simulink model "ACC_Main"  (R2025a)
settings: Solver=VariableStepAuto  StopTime=30
PostLoadFcn:
  | accRoot = fileparts(get_param('ACC_Main','FileName'));
  | addpath(accRoot, fullfile(accRoot,'models'), fullfile(accRoot,'scripts'));
  | run(fullfile(accRoot,'scripts','acc_init_setup.m'));
  | clear accRoot
undefined symbols (not defined in the file): D_followBlend_m, D_safe, k_closing
settings Model: Creator=Quang Huy  LastModifiedBy=ASUS
settings DebuggingCC: UnconnectedInputMsg=warning  UnconnectedOutputMsg=warning  UnconnectedLineMsg=warning

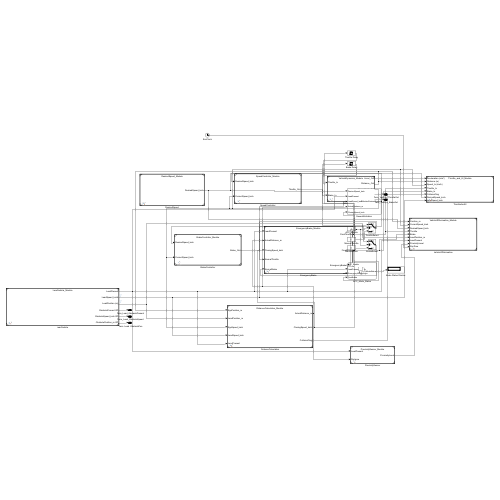
[thumbnail: Simulink's stored preview of the top-level diagram]
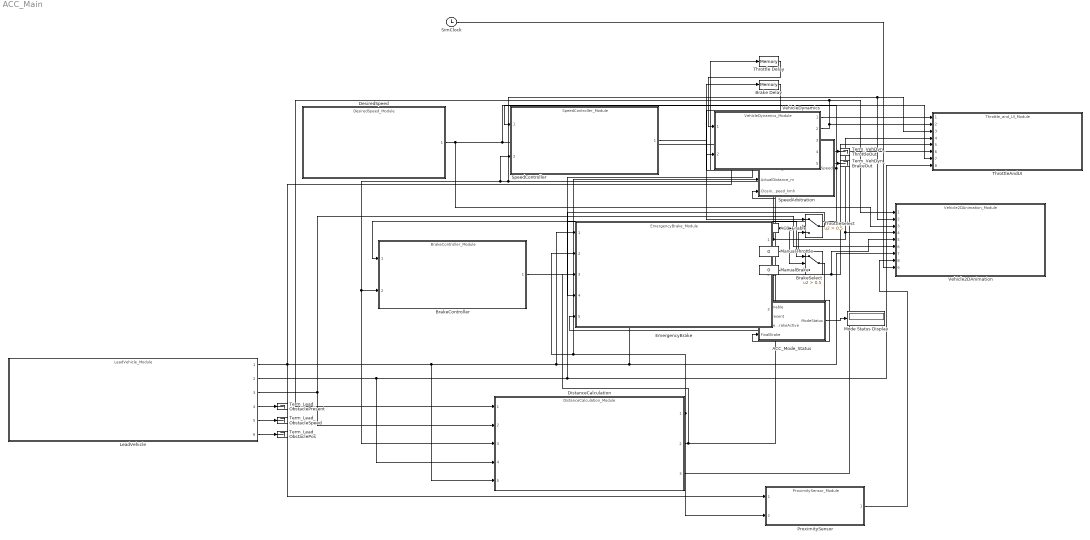
== system ACC_Main ==
  ACC_Enable : Constant  OutDataTypeStr=boolean
  ACC_Mode_Status : Stateflow chart  TreatAsAtomicUnit=on
  Brake Delay : Memory
  BrakeController : ModelReference  ModelNameDialog=BrakeController_Module.slx  SimulationMode=Normal  ModelReferenceVersion=3.0
  BrakeSelect : Switch  Criteria=u2 > Threshold  Threshold=0.5  SaturateOnIntegerOverflow=off  InputSameDT=off
  DesiredSpeed : ModelReference  ModelNameDialog=DesiredSpeed_Module.slx  SimulationMode=Normal  ModelReferenceVersion=3.0
  DistanceCalculation : ModelReference  ModelNameDialog=DistanceCalculation_Module.slx  SimulationMode=Normal  ModelReferenceVersion=3.0
  EmergencyBrake : ModelReference  ModelNameDialog=EmergencyBrake_Module.slx  SimulationMode=Normal  ModelReferenceVersion=3.0
  LeadVehicle : ModelReference  ModelNameDialog=LeadVehicle_Module.slx  SimulationMode=Normal  ModelReferenceVersion=3.2
  ManualBrake : Constant  Value=0
  ManualThrottle : Constant  Value=0  OutDataTypeStr=double
  Mode Status Display : Display
  ProximitySensor : ModelReference  ModelNameDialog=ProximitySensor_Module.slx  SimulationMode=Normal  ModelReferenceVersion=1.2
  SimClock : Clock
  SpeedArbitration : Subsystem
  SpeedController : ModelReference  ModelNameDialog=SpeedController_Module.slx  SimulationMode=Normal  ModelReferenceVersion=3.0
  Term_Lead_ObstaclePos : Terminator
  Term_Lead_ObstaclePresent : Terminator
  Term_Lead_ObstacleSpeed : Terminator
  Term_VehDyn_BrakeOut : Terminator
  Term_VehDyn_ThrottleOut : Terminator
  Throttle Delay : Memory
  ThrottleAndUI : ModelReference  ModelNameDialog=Throttle_and_UI_Module.slx  SimulationMode=Normal  ModelReferenceVersion=3.2
  ThrottleSelect : Switch  Criteria=u2 > Threshold  Threshold=0.5  SaturateOnIntegerOverflow=off  InputSameDT=off
  Vehicle2DAnimation : ModelReference  ModelNameDialog=Vehicle2DAnimation_Module.slx  SimulationMode=Normal  ModelReferenceVersion=3.1
  VehicleDynamics : ModelReference  ModelNameDialog=VehicleDynamics_Module.slx  SimulationMode=Normal  ModelReferenceVersion=3.0
  wires:
  DesiredSpeed/1 -> SpeedArbitration/1(DesiredSpeed_kmh), ThrottleAndUI/7, Vehicle2DAnimation/3
  LeadVehicle/3 -> DistanceCalculation/2, Vehicle2DAnimation/6
  LeadVehicle/2 -> SpeedArbitration/3(LeadSpeed_kmh), ThrottleAndUI/8, DistanceCalculation/4
  EmergencyBrake/1 -> Throttle Delay/1, ThrottleAndUI/4, Vehicle2DAnimation/4
  EmergencyBrake/2 -> Brake Delay/1, ThrottleAndUI/5, Vehicle2DAnimation/5, ACC_Mode_Status/4(FinalBrake)
  DistanceCalculation/2 -> EmergencyBrake/3, SpeedArbitration/5(ClosingSpeed_kmh)
  Throttle Delay/1 -> VehicleDynamics/1
  Brake Delay/1 -> VehicleDynamics/2
  DistanceCalculation/3 -> ThrottleAndUI/6
  SpeedArbitration/1(EffectiveDesiredSpeed) -> SpeedController/1, BrakeController/1
  SpeedController/1 -> ThrottleSelect/1
  ACC_Enable/1 -> ThrottleSelect/2, BrakeSelect/2, ACC_Mode_Status/1(ACC_Enable)
  ManualThrottle/1 -> ThrottleSelect/3
  ThrottleSelect/1 -> EmergencyBrake/4
  BrakeController/1 -> BrakeSelect/1
  ManualBrake/1 -> BrakeSelect/3
  BrakeSelect/1 -> EmergencyBrake/5
  EmergencyBrake/3 -> ACC_Mode_Status/3(EmergencyBrakeActive)
  ACC_Mode_Status/1(ModeStatus) -> Mode Status Display/1
  LeadVehicle/1 -> Vehicle2DAnimation/7, ACC_Mode_Status/2(LeadPresent), EmergencyBrake/1, DistanceCalculation/5, ProximitySensor/1, SpeedArbitration/2(LeadPresent)
  DistanceCalculation/1 -> EmergencyBrake/2, SpeedArbitration/4(ActualDistance_m), ProximitySensor/2
  ProximitySensor/1 -> Vehicle2DAnimation/8
  SimClock/1 -> Vehicle2DAnimation/9
  VehicleDynamics/2 -> Vehicle2DAnimation/1, DistanceCalculation/1, ThrottleAndUI/2
  VehicleDynamics/1 -> ThrottleAndUI/1
  VehicleDynamics/3 -> ThrottleAndUI/3, Vehicle2DAnimation/2, DistanceCalculation/3, BrakeController/2, SpeedController/2
  VehicleDynamics/4 -> Term_VehDyn_ThrottleOut/1
  VehicleDynamics/5 -> Term_VehDyn_BrakeOut/1
  LeadVehicle/4 -> Term_Lead_ObstaclePresent/1
  LeadVehicle/5 -> Term_Lead_ObstacleSpeed/1
  LeadVehicle/6 -> Term_Lead_ObstaclePos/1

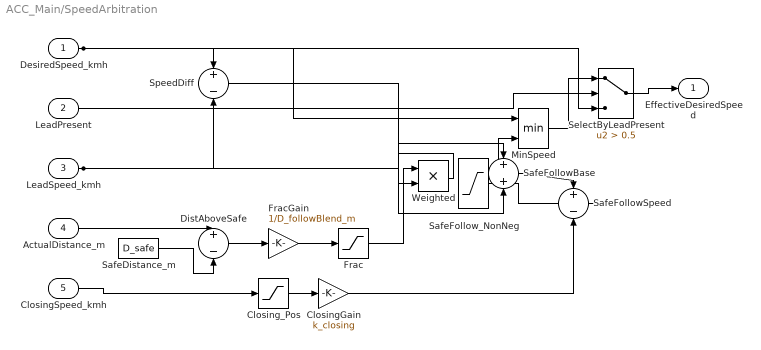
== system ACC_Main/SpeedArbitration ==
  DesiredSpeed_kmh : Inport
  LeadPresent : Inport  Port=2
  LeadSpeed_kmh : Inport  Port=3
  ActualDistance_m : Inport  Port=4
  ClosingSpeed_kmh : Inport  Port=5
  ClosingGain : Gain  Gain=k_closing
  Closing_Pos : Saturate  UpperLimit=inf  LowerLimit=0
  DistAboveSafe : Sum  Inputs=+-
  Frac : Saturate  UpperLimit=1  LowerLimit=0
  FracGain : Gain  Gain=1/D_followBlend_m
  MinSpeed : MinMax  Inputs=2
  SafeDistance_m : Constant  Value=D_safe
  SafeFollowBase : Sum
  SafeFollowSpeed : Sum  Inputs=+-
  SafeFollow_NonNeg : Saturate  UpperLimit=inf  LowerLimit=0
  SelectByLeadPresent : Switch  Criteria=u2 > Threshold  Threshold=0.5  SaturateOnIntegerOverflow=off  InputSameDT=off
  SpeedDiff : Sum  Inputs=+-
  Weighted : Product
  EffectiveDesiredSpeed : Outport
  wires:
  SafeDistance_m/1 -> DistAboveSafe/2
  ActualDistance_m/1 -> DistAboveSafe/1
  DistAboveSafe/1 -> FracGain/1
  ClosingSpeed_kmh/1 -> Closing_Pos/1
  Closing_Pos/1 -> ClosingGain/1
  LeadSpeed_kmh/1 -> SpeedDiff/2, SafeFollowBase/1
  ClosingGain/1 -> SafeFollowSpeed/2
  DesiredSpeed_kmh/1 -> MinSpeed/1, SelectByLeadPresent/3, SpeedDiff/1
  SafeFollow_NonNeg/1 -> MinSpeed/2
  MinSpeed/1 -> SelectByLeadPresent/1
  LeadPresent/1 -> SelectByLeadPresent/2
  SelectByLeadPresent/1 -> EffectiveDesiredSpeed/1
  FracGain/1 -> Frac/1
  Frac/1 -> Weighted/1
  SpeedDiff/1 -> Weighted/2
  Weighted/1 -> SafeFollowBase/2
  SafeFollowBase/1 -> SafeFollowSpeed/1
  SafeFollowSpeed/1 -> SafeFollow_NonNeg/1

== stateflow chart ACC_Main/ACC_Mode_Status ==
  state Off
    entry: ModeStatus = 0;
  state On
    during:
    if EmergencyBrakeActive
    ModeStatus = 4;
    elseif FinalBrake > 0
    ModeStatus = 3;
    elseif LeadPresent
    ModeStatus = 2;
    else
    ModeStatus = 1;
    end
  On -> Off : [~ACC_Enable]
  (default) -> Off
  Off -> On : [ACC_Enable]
  data: ACC_Enable input boolean; LeadPresent input boolean; EmergencyBrakeActive input boolean; FinalBrake input double; ModeStatus output uint8
